simulink model "SimOFDM_Total_Func_RS_116"  (R2022b)
settings: Solver=VariableStepAuto  StartTime=0.0  StopTime=inf  RelTol=1e-3
undefined symbols (not defined in the file): bits, doppler, rsgenpoly
libraries: commdigbbndam3 x4, commsink2 x3, dspindex x3, commofdm x3, commchan3 x2, commblkcod2 x2, commblkintrlv2 x2, commrandsrc3 x1
settings Model: Creator=v-c  LastModifiedBy=v-c

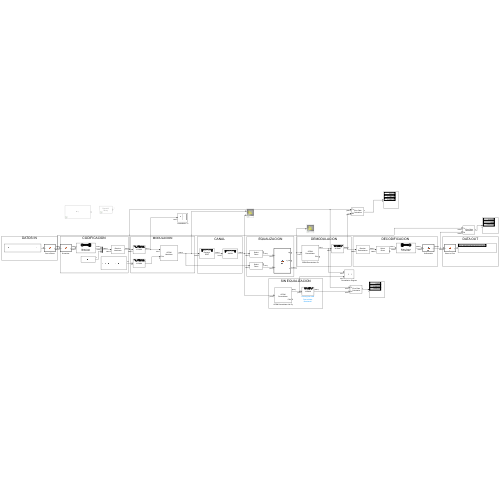
[thumbnail: Simulink's stored preview of the top-level diagram]
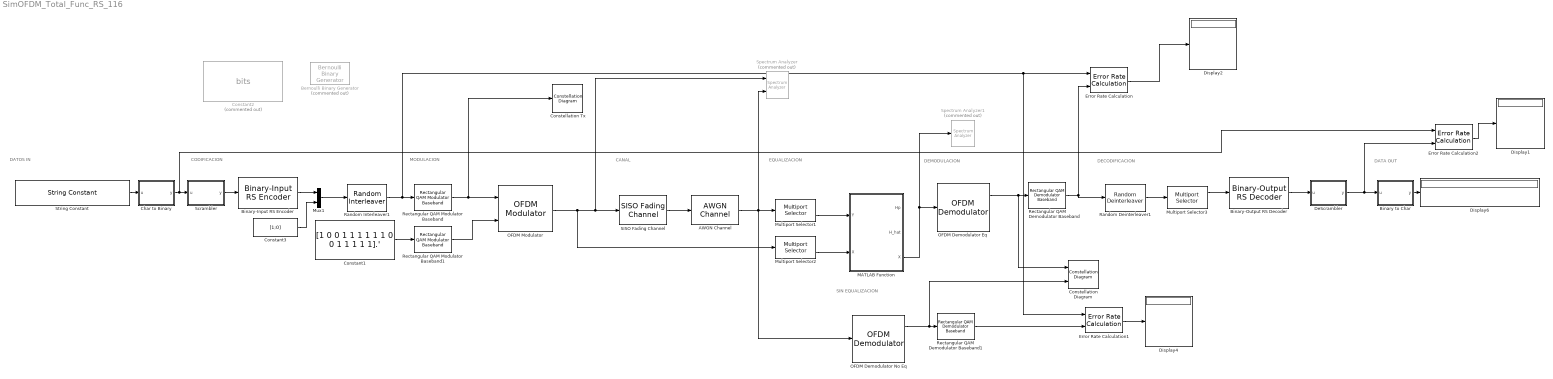
== system SimOFDM_Total_Func_RS_116 ==
  note: DATOS IN
  note: CODIFICACION
  note: MODULACION
  note: CANAL
  note: EQUALIZACION
  note: SIN EQUALIZACION
  note: DEMODULACION
  note: DECODIFICACION
  note: DATA OUT
  AWGN Channel : commchan3/AWGN Channel  InputProcessing=Columns as channels (frame based)  seed=67  noiseMode="Signal to noise ratio  (SNR)"  EbNodB=10  EsNodB=10  SNRdB=55  bitsPerSym=1  Ps=1  Tsym=1  variance=1
  Bernoulli Binary Generator : commrandsrc3/Bernoulli Binary Generator  Commented=on  ProbabilityOfZero=0.5  SeedSource=Auto  Seed=0  SampleTime=1  SamplesPerFrame=95*4  OutputDataType=double  SimulateUsing=Interpreted execution
  Binary to Char : MATLAB Function  TreatAsAtomicUnit=on
  Binary-Input RS Encoder : commblkcod2/Binary-Input RS Encoder  n=63  k=40  specShortening=off  shortenedK=3  specGenPoly=off  genPoly=rsgenpoly(7, 3, [], [], 'double')  specPrimPoly=off  prPoly='X^3 + X + 1'  specPuncture=off  punctVec=[ones(2,1); zeros(2,1)]  outDType=Same as input
  Binary-Output RS Decoder : commblkcod2/Binary-Output RS Decoder  n=63  k=40  specShortening=off  shortenedK=3  specGenPoly=off  genPoly=rsgenpoly(7, 3, [], [], 'double')  specPrimPoly=off  prPoly='X^3 + X + 1'  specPuncture=off  punctVec=[ones(2,1); zeros(2,1)]  specErasurePort=off  showNumErr=off  outDType=Same as input
  Char to Binary : MATLAB Function  TreatAsAtomicUnit=on
  Constant1 : Constant  Value=[1 0 0 1 1 1 1 1 1 0 0 1 1 1 1 1].'
  Constant2 : Constant  Commented=on  Value=bits  SampleTime=1
  Constant3 : Constant  Value=[1;0]
  Constellation Diagram : ConstellationDiagram  NumInputPorts=2  WindowPosition=[880.000000,78.000000,600.000000,600.000000,]  ScopeFrameLocation=window  ReferenceConstellation="{[16-QAM][0.7071+0.7071i          -0.7071+0.7071i          -0.7071-0.7071i            0.707-0.7071i]}"  ShowLegend=on
  Constellation Tx : ConstellationDiagram  WindowPosition=[32.000000,11.000000,600.000000,600.000000,]  ScopeFrameLocation=window
  DeScrambler : MATLAB Function  TreatAsAtomicUnit=on
  Display{1..2,4,6} (4 alike) : Display
  Error Rate Calculation : commsink2/Error Rate Calculation  N=0  st_delay=0  cp_mode=Entire frame  subframe=[]  PMode=Port  WsName=ErrorVec  RsMode2=off  stop=off  numErr=100  maxBits=1e6
      settings: LibrarySourceBlock=|
      | commhdlsink/Error Rate
      | Calculation
  Error Rate Calculation1 : commsink2/Error Rate Calculation  N=0  st_delay=0  cp_mode=Entire frame  subframe=[]  PMode=Port  WsName=ErrorVec  RsMode2=off  stop=off  numErr=100  maxBits=1e6
      settings: LibrarySourceBlock=|
      | commhdlsink/Error Rate
      | Calculation
  Error Rate Calculation2 : commsink2/Error Rate Calculation  N=0  st_delay=0  cp_mode=Entire frame  subframe=[]  PMode=Port  WsName=ErrorVec  RsMode2=off  stop=off  numErr=100  maxBits=1e6
  MATLAB Function : MATLAB Function  TreatAsAtomicUnit=on
  Multiport Selector1 : dspindex/Multiport Selector  rowsOrCols=Rows  idxCellArray={ 1:12,13:128}  idxErrMode=Clip Index
  Multiport Selector2 : dspindex/Multiport Selector  rowsOrCols=Rows  idxCellArray={ 1:12,13:128}  idxErrMode=Clip Index
  Multiport Selector3 : dspindex/Multiport Selector  rowsOrCols=Rows  idxCellArray={ 1:378, 379:380}  idxErrMode=Clip Index
  Mux1 : Mux  Inputs=2
  OFDM Demodulator Eq : commofdm/OFDM Demodulator  StatePerturbationForJacobian=1.0e-05  FFTLength=116  NumGuardBandCarriers=[8;8]  RemoveDCCarrier=on  PilotOutputPort=on  PilotCarrierIndices=[23;39;67;82]  CyclicPrefixLength=0  NumSymbols=1  NumReceiveAntennas=1  SimulateUsing=Interpreted execution
  OFDM Demodulator No Eq : commofdm/OFDM Demodulator  StatePerturbationForJacobian=1.0e-05  FFTLength=116  NumGuardBandCarriers=[8;8]  RemoveDCCarrier=on  PilotOutputPort=on  PilotCarrierIndices=[23;39;67;82]  CyclicPrefixLength=12  NumSymbols=1  NumReceiveAntennas=1  SimulateUsing=Interpreted execution
  OFDM Modulator : commofdm/OFDM Modulator  StatePerturbationForJacobian=1.0e-05  FFTLength=116  NumGuardBandCarriers=[8;8]  InsertDCNull=on  PilotInputPort=on  PilotCarrierIndices=[23;39;67;82]  CyclicPrefixLength=12  Windowing=off  WindowLength=1  NumSymbols=1  NumTransmitAntennas=1  SimulateUsing=Interpreted execution
  Random Deinterleaver1 : commblkintrlv2/Random Deinterleaver  StatePerturbationForJacobian=1.0e-05  N=380  seed=12345
  Random Interleaver1 : commblkintrlv2/Random Interleaver  StatePerturbationForJacobian=1.0e-05  N=380  seed=12345
  Rectangular QAM Demodulator Baseband : commdigbbndam3/Rectangular QAM Demodulator Baseband  M=16  OutType=Bit  DecType=Hard decision  VarSource=Dialog  Variance=1  Dec=Gray  Mapping=[0:15]  PowType=Average Power  MinDist=2  AvgPow=1  PeakPow=1  Ph=0  outDtype1=Inherit via internal rule  outDtype2=Inherit via internal rule  derotateFactorWordLen=16  derotateFactorDataTypeStr=Inherit: Same word length as input  derotateFactorLastDataTypeStr=Inherit: Same word length as input  denormFactorWordLen=16  denormFactorDataTypeStr=Inherit: Same word length as input  denormFactorLastDataTypeStr=Inherit: Same word length as input  prodOutWordLen=32  prodOutOverflowMode=Wrap  prodOutRoundingMode=Floor  prodOutOvFlMode=off  prodOutOvFlModeLastStrValue=off  sumWordLen=32
      settings: LibrarySourceBlock=|
      | commhdldigbbndam/Rectangular QAM
      | Demodulator
      | Baseband
  Rectangular QAM Demodulator Baseband1 : commdigbbndam3/Rectangular QAM Demodulator Baseband  M=16  OutType=Bit  DecType=Hard decision  VarSource=Dialog  Variance=1  Dec=Gray  Mapping=[0:15]  PowType=Average Power  MinDist=2  AvgPow=1  PeakPow=1  Ph=0  outDtype1=Inherit via internal rule  outDtype2=Inherit via internal rule  derotateFactorWordLen=16  derotateFactorDataTypeStr=Inherit: Same word length as input  derotateFactorLastDataTypeStr=Inherit: Same word length as input  denormFactorWordLen=16  denormFactorDataTypeStr=Inherit: Same word length as input  denormFactorLastDataTypeStr=Inherit: Same word length as input  prodOutWordLen=32  prodOutOverflowMode=Wrap  prodOutRoundingMode=Floor  prodOutOvFlMode=off  prodOutOvFlModeLastStrValue=off  sumWordLen=32
      settings: LibrarySourceBlock=|
      | commhdldigbbndam/Rectangular QAM
      | Demodulator
      | Baseband
  Rectangular QAM Modulator Baseband : commdigbbndam3/Rectangular QAM Modulator Baseband  M=16  InType=Bit  Enc=Gray  Mapping=[0:15]  PowType=Average Power  MinDist=2  AvgPow=1  PeakPow=1  Ph=0  outDtype=double  outWordLen=16  outUDDataType=sfix(16)  outFracLenMode=Best precision  outFracLen=15  outDataTypeStr=double  outLastDataTypeStr=double
      settings: LibrarySourceBlock=|
      | commhdldigbbndam/Rectangular QAM
      | Modulator
      | Baseband
  Rectangular QAM Modulator Baseband1 : commdigbbndam3/Rectangular QAM Modulator Baseband  M=16  InType=Bit  Enc=Gray  Mapping=[0:15]  PowType=Average Power  MinDist=2  AvgPow=1  PeakPow=1  Ph=0  outDtype=double  outWordLen=16  outUDDataType=sfix(16)  outFracLenMode=Best precision  outFracLen=15  outDataTypeStr=double  outLastDataTypeStr=double
      settings: LibrarySourceBlock=|
      | commhdldigbbndam/Rectangular QAM
      | Modulator
      | Baseband
  SISO Fading Channel : commchan3/SISO Fading Channel  InheritSampleRate=on  SampleRate=1  PathDelays=0.5e-09*[0 0.2000 0.4000 0.8000]  AveragePathGains=[0 -3 -6 -9]  NormalizePathGains=on  FadingDistribution=Rayleigh  KFactor=3  DirectPathDopplerShift=0  DirectPathInitialPhase=0  MaximumDopplerShift=270  DopplerSpectrum=doppler('Jakes')  RandomStream=mt19937ar with seed  Seed=40  PathGainsOutputPort=off  ChannelFilterDelayOutputPort=off  SimulateUsing=Interpreted execution  Visualization=Off  PathsForDopplerDisplay=1  SamplesToDisplay=25%
  Scrambler : MATLAB Function  TreatAsAtomicUnit=on
  Spectrum Analyzer : SpectrumAnalyzer  Commented=on  NumInputPorts=2
  Spectrum Analyzer1 : SpectrumAnalyzer  Commented=on
  String Constant : StringConstant  String="\"Kron MundoHola MundoHola Mundo\""
  wires:
  Constant1/1 -> Rectangular QAM Modulator Baseband1/1
  Rectangular QAM Modulator Baseband1/1 -> OFDM Modulator/2
  Rectangular QAM Modulator Baseband/1 -> OFDM Modulator/1, Constellation Tx/1
  OFDM Modulator/1 -> SISO Fading Channel/1, Spectrum Analyzer/1, Multiport Selector2/1
  Error Rate Calculation/1 -> Display2/1
  OFDM Demodulator Eq/1 -> Constellation Diagram/1, Rectangular QAM Demodulator Baseband/1
  SISO Fading Channel/1 -> AWGN Channel/1
  Rectangular QAM Demodulator Baseband1/1 -> Error Rate Calculation1/2
  OFDM Demodulator No Eq/1 -> Constellation Diagram/2, Rectangular QAM Demodulator Baseband1/1
  Error Rate Calculation1/1 -> Display4/1
  Multiport Selector1/2 -> MATLAB Function/1(Y)
  Multiport Selector2/2 -> MATLAB Function/2("X ")
  MATLAB Function/3(X) -> OFDM Demodulator Eq/1, Spectrum Analyzer1/1
  Random Interleaver1/1 -> Rectangular QAM Modulator Baseband/1, Error Rate Calculation/1, Error Rate Calculation1/1
  String Constant/1 -> Char to Binary/1(u)
  Binary-Input RS Encoder/1 -> Mux1/1
  Scrambler/1(y) -> Binary-Input RS Encoder/1
  Mux1/1 -> Random Interleaver1/1
  Constant3/1 -> Mux1/2
  Multiport Selector3/1 -> Binary-Output RS Decoder/1
  Binary to Char/1(y) -> Display6/1
  Random Deinterleaver1/1 -> Multiport Selector3/1
  Binary-Output RS Decoder/1 -> DeScrambler/1(u)
  DeScrambler/1(y) -> Binary to Char/1(u), Error Rate Calculation2/2
  Rectangular QAM Demodulator Baseband/1 -> Random Deinterleaver1/1, Error Rate Calculation/2
  Char to Binary/1(y) -> Error Rate Calculation2/1, Scrambler/1(u)
  AWGN Channel/1 -> Spectrum Analyzer/2, Multiport Selector1/1, OFDM Demodulator No Eq/1
  Error Rate Calculation2/1 -> Display1/1

== matlab function SimOFDM_Total_Func_RS_116/Char to Binary ==
  settings: updateMethod=DISCRETE  sampleTime=1/(15e3)
  data: u input; y output size=[240 1]
function y = fcn(u)
Txt = char(u);
unicode = uint8 (Txt); %conversion para 8 bits
Bits = zeros(240,1);cont = 1;
for i = 1 : 30
    Aux1 = dec2bin(unicode(1,i),8);
    for j = 1: 8
        Bits(cont,1) = bin2dec(Aux1 (1,j));
        cont = cont +1;
    end
end
y = Bits;

== matlab function SimOFDM_Total_Func_RS_116/MATLAB Function ==
  data: Y input size=[116 1]; Hp output size=[4 1]; X input size=[116 1]; H_hat output; X output size=[116 1]
function [Hp, H_hat,X] = fcn(Y,X)
IndxPilot = [23;39;67;82]; %[12; 26; 40; 54]-6; 

%calculando la FFT
Yp = Y(IndxPilot);
Xp = X(IndxPilot);
%matriz piloit
Xp =  diag(Xp);
Hp = inv(Xp)*Yp;
H_hat = (interp1 (IndxPilot,Hp,1:116,'spline','extrap')).';
X = Y./H_hat;
[Hp];%= [0;0;0;0];

== matlab function SimOFDM_Total_Func_RS_116/Scrambler ==
  data: u input; y output
function y = fcn(u)
scramInit = 25;
scrambledData = wlanScramble(u,scramInit);
y = scrambledData;

== matlab function SimOFDM_Total_Func_RS_116/Binary to Char ==
  data: u input size=[240 1]; y output
function y = fcn(u)
aux2 = '00000000';
%conversion en unicode
unicodeR = zeros(1,30);
cont = 0;
for j = 1: 30
    for i = 1+cont: 8 + cont
        aux2(1,i-cont) = dec2bin (u(i,1));   
    end 
    cont = cont + 8;
    unicodeR(1,j) = bin2dec (aux2);
end
TxTR = convertCharsToStrings(char(unicodeR));
y = TxTR;

== matlab function SimOFDM_Total_Func_RS_116/DeScrambler ==
  data: u input; y output
function y = fcn(u)
scramInit = 25;
descrambledData = wlanScramble(u,scramInit);
y = descrambledData;
